simulink model "airdrag"  (R2024b)
settings: Solver=FixedStepAuto  StartTime=0.0  StopTime=10.0  FixedStep=0.1  RelTol=1e-3
values from neighbouring files (symbols this model uses):
  Ar = [6e-2; 6e-2; 6e-2; 6e-2; 4e-2; 4e-2; 12e-2; 12e-2; 12e-2; 12e-2]    [LabsDCM.m]    (also in Srp_Lab7.m; airdrag.m)
  Cd = [2.4631105; 2.1042609; 2.4631105; 2.1042609; 1.4675356; 1.4675356; 2.547683; 2.547683; 2.547683; 2.547683]    [airdrag.m]
  J = diag([Ix Iy Iz])    [LabsDCM.m]    (also in Srp_Lab7.m; airdrag.m)
  n = sqrt(G*M/(R^3))    [LabsDCM.m]    (also in Srp_Lab7.m; airdrag.m)
  N_B = [ 1,  0,  0 ... (first row only)    [LabsDCM.m]    (also in Srp_Lab7.m; airdrag.m)
  r_Fi = [ ... (first row only)    [LabsDCM.m]    (also in Srp_Lab7.m; airdrag.m)
  rho = rho_0 * exp(-(h-h0)/H)    [airdrag.m]
  W0 = [0.45 0.52 0.55]    [LabsDCM.m]    (also in Srp_Lab7.m; airdrag.m)
  w_0e = 0.000072921    (= 7.2921e-05)    [airdrag.m]
undefined symbols (not defined in the file or in its folder): a, e, i
libraries: matrix_library x3, dspmathops x1
settings Model: Creator=User  LastModifiedBy=User

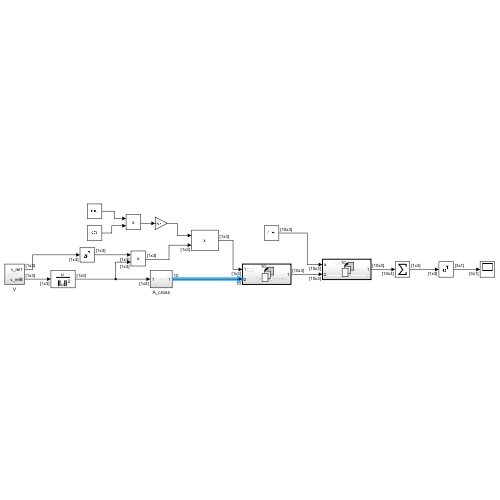
[thumbnail: Simulink's stored preview of the top-level diagram]
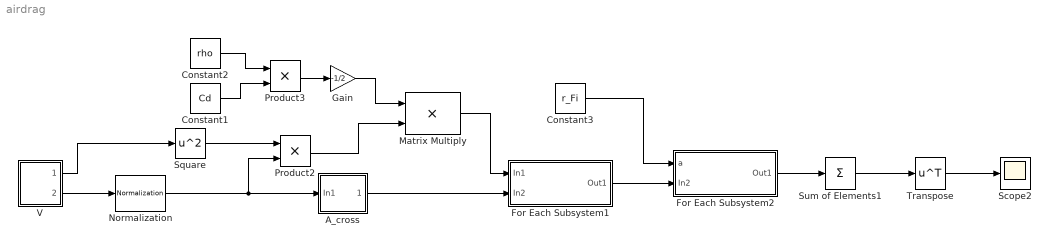
== system airdrag ==
  A_cross : Subsystem
  Constant1 : Constant  Value=Cd
  Constant2 : Constant  Value=rho
  Constant3 : Constant  Value=r_Fi
  For Each Subsystem1 : Subsystem  TreatAsAtomicUnit=on
  For Each Subsystem2 : Subsystem  TreatAsAtomicUnit=on
  Gain : Gain  Gain=-1/2
  Matrix Multiply : Product
  Normalization : dspmathops/Normalization  NormType=Squared 2-norm  Bias=1e-10  NormOver=Each column  Dimension=1  roundingMode=Floor  overflowMode=off  accumDataTypeStr=Inherit: Same as product output  accumLastDataTypeStr=Inherit: Same as product output  outputDataTypeStr=Inherit: Same as product output  outputMin=[]  outputMax=[]  outputLastDataTypeStr=Inherit: Same as product output
  Product2 : Product
  Product3 : Product
  Scope2 : Scope
  Square : Math  Operator=square
  Sum of Elements1 : Sum  Inputs=+  CollapseMode=Specified dimension
  Transpose : Math  Operator=transpose
  V : Subsystem
  wires:
  Normalization/1 -> A_cross/1(In1), Product2/2
  Product2/1 -> Matrix Multiply/2
  Constant1/1 -> Product3/2
  Square/1 -> Product2/1
  Constant2/1 -> Product3/1
  Product3/1 -> Gain/1
  Gain/1 -> Matrix Multiply/1
  Constant3/1 -> For Each Subsystem2/1(a)
  V/1(v_rel1) -> Square/1
  V/2(v_relB) -> Normalization/1
  For Each Subsystem2/1(Out1) -> Sum of Elements1/1
  Sum of Elements1/1 -> Transpose/1
  Transpose/1 -> Scope2/1
  Matrix Multiply/1 -> For Each Subsystem1/1(In1)
  A_cross/1(Out1) -> For Each Subsystem1/2(In2)
  For Each Subsystem1/1(Out1) -> For Each Subsystem2/2(In2)

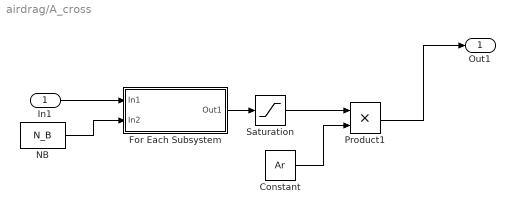
== system airdrag/A_cross ==
  In1 : Inport
  Constant : Constant  Value=Ar
  For Each Subsystem : Subsystem  TreatAsAtomicUnit=on
  NB : Constant  Value=N_B
  Product1 : Product
  Saturation : Saturate  UpperLimit=inf  LowerLimit=0
  Out1 : Outport
  wires:
  In1/1 -> For Each Subsystem/1(In1)
  Product1/1 -> Out1/1
  Saturation/1 -> Product1/1
  Constant/1 -> Product1/2
  NB/1 -> For Each Subsystem/2(In2)
  For Each Subsystem/1(Out1) -> Saturation/1

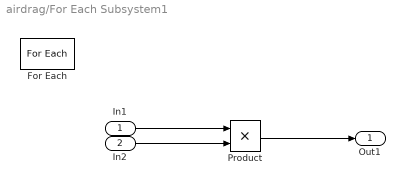
== system airdrag/For Each Subsystem1 ==
  In1 : Inport
  In2 : Inport  Port=2  Partition=on  PartitionDimension=1  PartitionWidth=1  PartitionOffset=0
  For Each : ForEach  DisableCoverage=on  SpecifiedNumIters=10
  Product : Product
  Out1 : Outport  ConcatenationDimension=1
  wires:
  In1/1 -> Product/1
  Product/1 -> Out1/1
  In2/1 -> Product/2

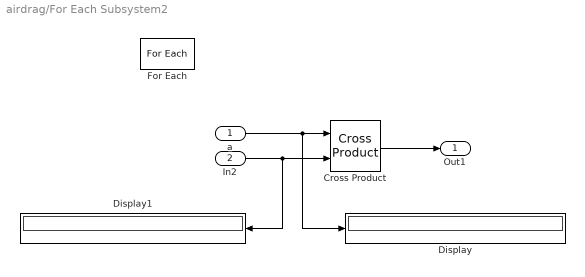
== system airdrag/For Each Subsystem2 ==
  a : Inport  Partition=on  PartitionDimension=1  PartitionWidth=1  PartitionOffset=0
  In2 : Inport  Port=2  Partition=on  PartitionDimension=1  PartitionWidth=1  PartitionOffset=0
  Cross Product : matrix_library/Cross Product
  Display : Display
  Display1 : Display
  For Each : ForEach  DisableCoverage=on
  Out1 : Outport  ConcatenationDimension=1
  wires:
  a/1 -> Display/1, Cross Product/1
  In2/1 -> Display1/1, Cross Product/2
  Cross Product/1 -> Out1/1

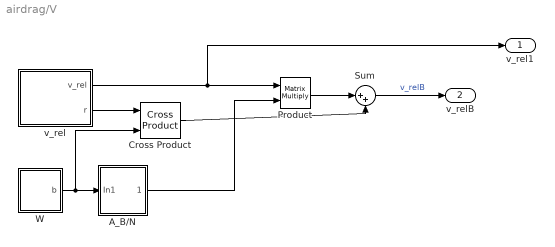
== system airdrag/V ==
  A_B/N : Subsystem
  Cross Product : matrix_library/Cross Product
  Product : Product  Multiplication=Matrix(*)
  Sum : Sum  Inputs=|++
  W : Subsystem
  v_rel : Subsystem
  v_rel1 : Outport
  v_relB : Outport  Port=2
  wires:
  Product/1 -> Sum/1
  v_rel/2(r) -> Cross Product/1
  Cross Product/1 -> Sum/2
  W/1(b) -> Cross Product/2, A_B/N/1(In1)
  A_B/N/1(Out1) -> Product/2
  v_rel/1(v_rel) -> v_rel1/1, Product/1
  Sum/1 -> v_relB/1  "v_relB"

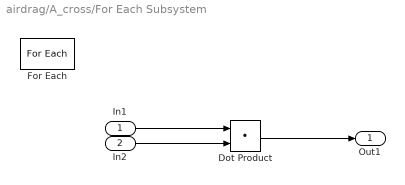
== system airdrag/A_cross/For Each Subsystem ==
  In1 : Inport
  In2 : Inport  Port=2  Partition=on  PartitionDimension=1  PartitionWidth=1  PartitionOffset=0
  Dot Product : DotProduct  OutDataTypeStr=Inherit: Inherit via internal rule
  For Each : ForEach  DisableCoverage=on  SpecifiedNumIters=10
  Out1 : Outport  ConcatenationDimension=1
  wires:
  In1/1 -> Dot Product/1
  Dot Product/1 -> Out1/1
  In2/1 -> Dot Product/2

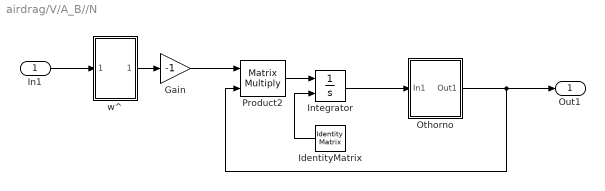
== system airdrag/V/A_B//N ==
  In1 : Inport
  Gain : Gain  Gain=-1
  IdentityMatrix : IdentityMatrix  OutputDimensions=3
  Integrator : Integrator  InitialConditionSource=external
  Othorno : Subsystem
  Product2 : Product  Multiplication=Matrix(*)
  w^ : Subsystem
  Out1 : Outport
  wires:
  Gain/1 -> Product2/1
  Integrator/1 -> Othorno/1(In1)
  Othorno/1(Out1) -> Out1/1, Product2/2
  In1/1 -> w^/1(In1)
  w^/1(Out1) -> Gain/1
  Product2/1 -> Integrator/1
  IdentityMatrix/1 -> Integrator/2

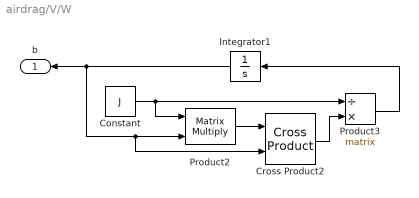
== system airdrag/V/W ==
  Constant : Constant  Value=J
  Cross Product2 : matrix_library/Cross Product
  Integrator1 : Integrator  InitialCondition=W0
  Product2 : Product  Multiplication=Matrix(*)
  Product3 : Product  Inputs=/*  Multiplication=Matrix(*)
  b : Outport
  wires:
  Cross Product2/1 -> Product3/2
  Integrator1/1 -> Cross Product2/2, Product2/2, b/1
  Constant/1 -> Product2/1, Product3/1
  Product2/1 -> Cross Product2/1
  Product3/1 -> Integrator1/1

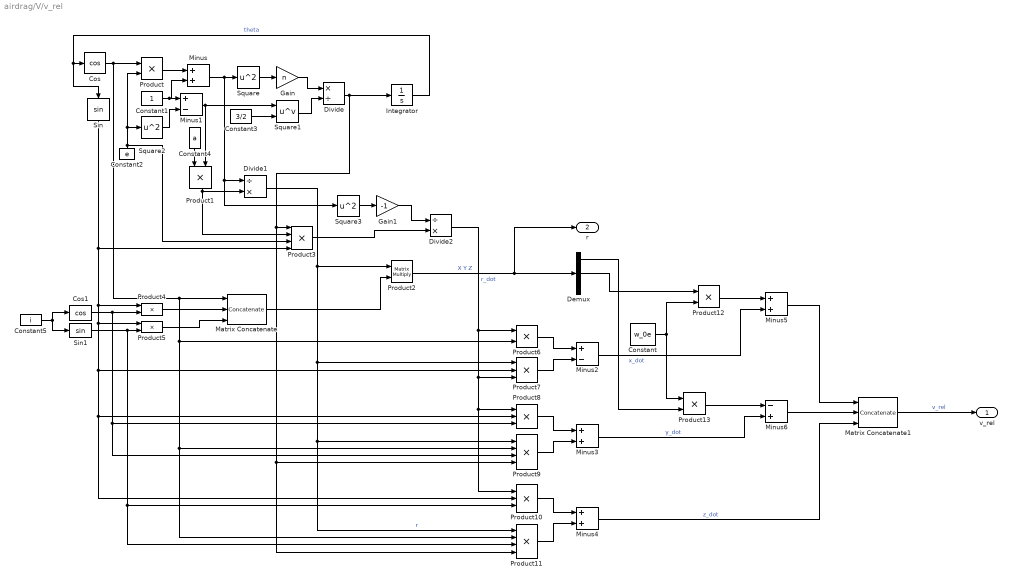
== system airdrag/V/v_rel ==
  Constant : Constant  Value=w_0e
  Constant1 : Constant
  Constant2 : Constant  Value=e
  Constant3 : Constant  Value=3/2
  Constant4 : Constant  Value=a
  Constant5 : Constant  Value=i
  Cos : Trigonometry  Operator=cos
  Cos1 : Trigonometry  Operator=cos
  Demux : Demux  Outputs=3
  Divide : Product  Inputs=*/
  Divide1 : Product  Inputs=/*
  Divide2 : Product  Inputs=/*
  Gain : Gain  Gain=n
  Gain1 : Gain  Gain=-1
  Integrator : Integrator
  Matrix Concatenate : Concatenate  NumInputs=3  Mode=Multidimensional array  ConcatenateDimension=2
  Matrix Concatenate1 : Concatenate  NumInputs=3  Mode=Multidimensional array  ConcatenateDimension=2
  Minus{,3..5} (4 alike) : Sum
  Minus1 : Sum  Inputs=+-
  Minus2 : Sum  Inputs=+-
  Minus6 : Sum  Inputs=-+
  Product{,1,4..6,12..13} (7 alike) : Product
  Product10 : Product  Inputs=3
  Product11 : Product  Inputs=4
  Product2 : Product  Multiplication=Matrix(*)
  Product3 : Product  Inputs=4
  Product7 : Product  Inputs=3
  Product8 : Product  Inputs=3
  Product9 : Product  Inputs=4
  Sin : Trigonometry
  Sin1 : Trigonometry
  Square : Math  Operator=square
  Square1 : Math  Operator=pow
  Square2 : Math  Operator=square
  Square3 : Math  Operator=square
  v_rel : Outport
  r : Outport  Port=2
  wires:
  Cos1/1 -> Product4/2, Product9/3, Product8/3
  Product8/1 -> Minus3/1
  Sin/1 -> Product10/2, Product8/2, Product7/2, Product5/1, Product4/1, Product3/4
  Square/1 -> Gain/1
  Cos/1 -> Matrix Concatenate/1, Product11/2, Product9/2, Product6/2, Product/1
  Divide/1 -> Integrator/1, Product11/4, Product9/4, Product3/1
  Product12/1 -> Minus5/1
  Minus1/1 -> Square1/1, Product1/2
  Divide2/1 -> Product7/3, Product10/1, Product8/1, Product6/1  "r_dot"
  Minus3/1 -> Minus6/2  "y_dot"
  Product13/1 -> Minus6/1
  Product10/1 -> Minus4/1
  Sin1/1 -> Product5/2, Product11/3, Product10/3
  Product9/1 -> Minus3/2
  Constant5/1 -> Cos1/1, Sin1/1
  Product7/1 -> Minus2/2
  Square3/1 -> Gain1/1
  Minus/1 -> Square3/1, Divide1/1, Square/1
  Minus6/1 -> Matrix Concatenate1/2
  Product6/1 -> Minus2/1
  Product11/1 -> Minus4/2
  Divide1/1 -> Product11/1, Product9/1, Product7/1, Product2/1  "r"
  Square1/1 -> Divide/2
  Constant2/1 -> Product3/3, Product/2, Square2/1
  Matrix Concatenate/1 -> Product2/2
  Square2/1 -> Minus1/2
  Product2/1 -> Demux/1, r/1  "X Y Z"
  Product5/1 -> Matrix Concatenate/3
  Gain/1 -> Divide/1
  Constant/1 -> Product12/2, Product13/1
  Demux/1 -> Product13/2
  Integrator/1 -> Sin/1, Cos/1  "theta"
  Demux/2 -> Product12/1
  Minus5/1 -> Matrix Concatenate1/1
  Product/1 -> Minus/1
  Constant3/1 -> Square1/2
  Product1/1 -> Product3/2, Divide1/2
  Product4/1 -> Matrix Concatenate/2
  Constant4/1 -> Product1/1
  Constant1/1 -> Minus/2, Minus1/1
  Minus2/1 -> Minus5/2  "x_dot"
  Product3/1 -> Divide2/2
  Gain1/1 -> Divide2/1
  Minus4/1 -> Matrix Concatenate1/3  "z_dot"
  Matrix Concatenate1/1 -> v_rel/1  "v_rel"

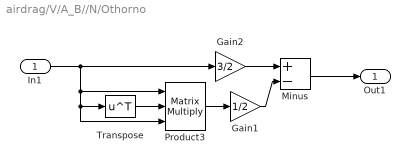
== system airdrag/V/A_B//N/Othorno ==
  In1 : Inport
  Gain1 : Gain  Gain=1/2
  Gain2 : Gain  Gain=3/2
  Minus : Sum  Inputs=+-
  Product3 : Product  Inputs=3  Multiplication=Matrix(*)
  Transpose : Math  Operator=transpose
  Out1 : Outport
  wires:
  Gain1/1 -> Minus/2
  Gain2/1 -> Minus/1
  In1/1 -> Product3/3, Transpose/1, Product3/1, Gain2/1
  Transpose/1 -> Product3/2
  Product3/1 -> Gain1/1
  Minus/1 -> Out1/1

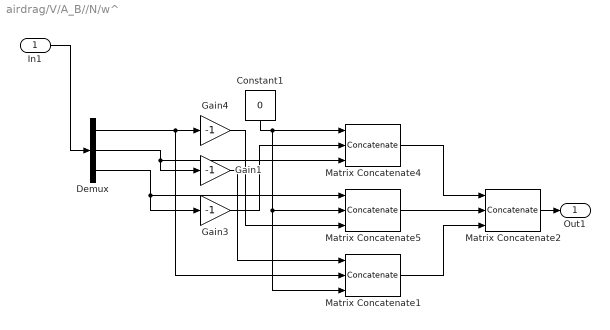
== system airdrag/V/A_B//N/w^ ==
  In1 : Inport
  Constant1 : Constant  Value=0
  Demux : Demux  Outputs=3
  Gain1 : Gain  Gain=-1
  Gain3 : Gain  Gain=-1
  Gain4 : Gain  Gain=-1
  Matrix Concatenate1 : Concatenate  NumInputs=3  Mode=Multidimensional array  ConcatenateDimension=2
  Matrix Concatenate2 : Concatenate  NumInputs=3  Mode=Multidimensional array
  Matrix Concatenate4 : Concatenate  NumInputs=3  Mode=Multidimensional array  ConcatenateDimension=2
  Matrix Concatenate5 : Concatenate  NumInputs=3  Mode=Multidimensional array  ConcatenateDimension=2
  Out1 : Outport
  wires:
  Matrix Concatenate1/1 -> Matrix Concatenate2/3
  Gain3/1 -> Matrix Concatenate4/2
  Constant1/1 -> Matrix Concatenate4/1, Matrix Concatenate5/2, Matrix Concatenate1/3
  Demux/3 -> Gain3/1, Matrix Concatenate5/1
  Demux/1 -> Gain4/1, Matrix Concatenate1/2
  Matrix Concatenate5/1 -> Matrix Concatenate2/2
  Demux/2 -> Gain1/1, Matrix Concatenate4/3
  Matrix Concatenate4/1 -> Matrix Concatenate2/1
  Gain4/1 -> Matrix Concatenate5/3
  Gain1/1 -> Matrix Concatenate1/1
  Matrix Concatenate2/1 -> Out1/1
  In1/1 -> Demux/1
